simulink model "calculate_thrust"  (R2026a)
settings: Solver=VariableStepAuto
libraries: robotcorelib x1
settings Model: Creator=eqtran103  LastModifiedBy=eqtran103

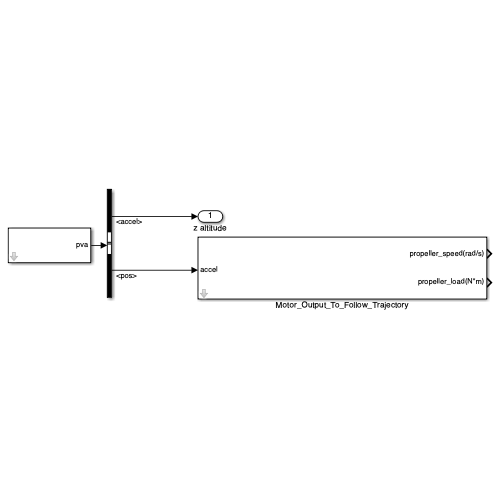
[thumbnail: Simulink's stored preview of the top-level diagram]
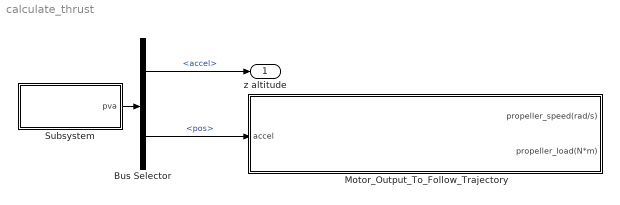
== system calculate_thrust ==
  Bus Selector : BusSelector  OutputSignals=accel,pos
  Motor_Output_To_Follow_Trajectory : Subsystem  mask{Parameter1=0}
  Subsystem : Subsystem  mask{SnapAmplitude=1, JerkCoupleWidth=26.942, TrajectoryTime=100, MaxAccel=1, LaunchTime=10}
  z altitude : Outport
  wires:
  Bus Selector/2 -> Motor_Output_To_Follow_Trajectory/1(accel)  "<pos>"
  Subsystem/1(pva) -> Bus Selector/1
  Bus Selector/1 -> z altitude/1  "<accel>"

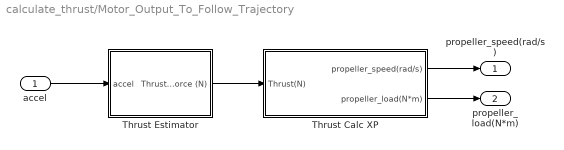
== system calculate_thrust/Motor_Output_To_Follow_Trajectory ==
  accel : Inport
  Thrust Calc XP : Subsystem  mask{L_C=0.02, L_to_D=10}
      mask prompts: L_C "Lift Coefficent (N/(rad/s)^2)"; L_to_D "Lift to Drag (m)"
  Thrust Estimator : Subsystem
  propeller_speed(rad/s) : Outport
  propeller_load(N*m) : Outport  Port=2
  wires:
  Thrust Calc XP/2(propeller_load(N*m)) -> propeller_load(N*m)/1
  accel/1 -> Thrust Estimator/1(accel)
  Thrust Calc XP/1(propeller_speed(rad/s)) -> propeller_speed(rad/s)/1
  Thrust Estimator/1(Thrust_Force (N)) -> Thrust Calc XP/1(Thrust(N))

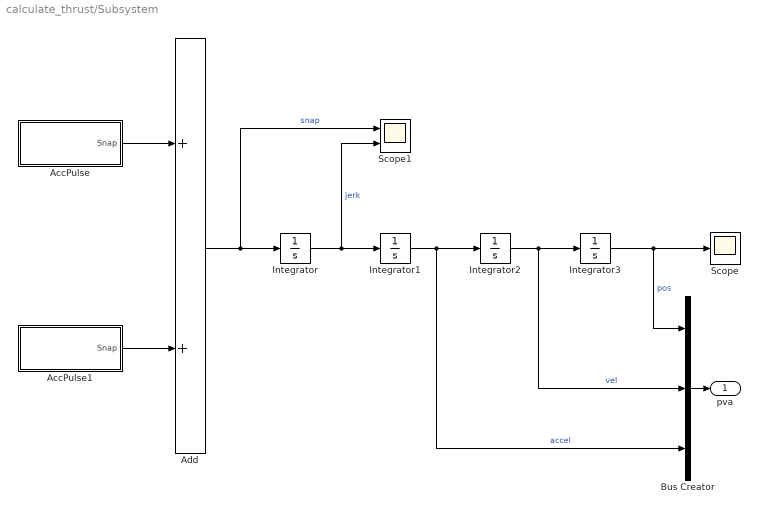
== system calculate_thrust/Subsystem ==
  AccPulse : Subsystem  mask{Amplitude=SnapAmplitude, Width=JerkCoupleWidth, StartTime=LaunchTime}
  AccPulse1 : Subsystem  mask{Amplitude=-SnapAmplitude, Width=JerkCoupleWidth, StartTime=TrajectoryTime - 2*JerkCoupleWidth}
  Add : Sum
  Bus Creator : BusCreator  Inputs=3
  Integrator{,1..3} (4 alike) : Integrator
  Scope : Scope
  Scope1 : Scope  NumInputPorts=2
  pva : Outport
  wires:
  AccPulse/1(Snap) -> Add/1
  AccPulse1/1(Snap) -> Add/2
  Add/1 -> Scope1/1, Integrator/1  "snap"
  Integrator/1 -> Scope1/2, Integrator1/1  "jerk"
  Integrator1/1 -> Bus Creator/3, Integrator2/1  "accel"
  Integrator2/1 -> Bus Creator/2, Integrator3/1  "vel"
  Integrator3/1 -> Bus Creator/1, Scope/1  "pos"
  Bus Creator/1 -> pva/1

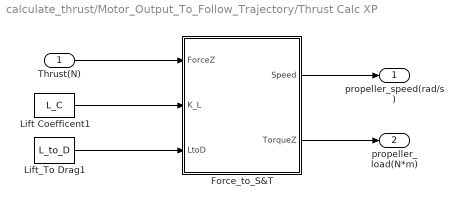
== system calculate_thrust/Motor_Output_To_Follow_Trajectory/Thrust Calc XP ==
  Thrust(N) : Inport
  Force_to_S&T : MATLAB Function  TreatAsAtomicUnit=on
  Lift Coefficent1 : Constant  Value=L_C
  Lift_To Drag1 : Constant  Value=L_to_D
  propeller_speed(rad/s) : Outport
  propeller_load(N*m) : Outport  Port=2
  wires:
  Thrust(N)/1 -> Force_to_S&T/1(ForceZ)
  Lift Coefficent1/1 -> Force_to_S&T/2(K_L)
  Lift_To Drag1/1 -> Force_to_S&T/3(LtoD)
  Force_to_S&T/2(TorqueZ) -> propeller_load(N*m)/1
  Force_to_S&T/1(Speed) -> propeller_speed(rad/s)/1

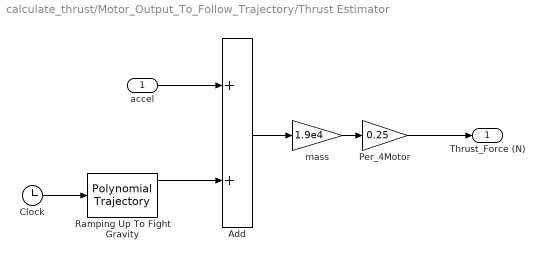
== system calculate_thrust/Motor_Output_To_Follow_Trajectory/Thrust Estimator ==
  accel : Inport
  Add : Sum
  Clock : Clock
  Per_4Motor : Gain  Gain=0.25
  Ramping Up To Fight Gravity : robotcorelib/Polynomial Trajectory  WaypointSource=Internal  Waypoints=[ 0, 9.8]  TimePoints=[ 0, 8]  TimeInterval=[ 1, 4 ]  Method=Cubic Polynomial  ParameterSource=Internal  VelocityBoundaryCondition=zeros( 1, 2 )  AccelerationBoundaryCondition=zeros( 2, 5 )  SimulateUsing=Interpreted execution
  mass : Gain  Gain=1.9e4
  Thrust_Force (N) : Outport
  wires:
  accel/1 -> Add/1
  mass/1 -> Per_4Motor/1
  Add/1 -> mass/1
  Per_4Motor/1 -> Thrust_Force (N)/1
  Clock/1 -> Ramping Up To Fight Gravity/1
  Ramping Up To Fight Gravity/1 -> Add/2

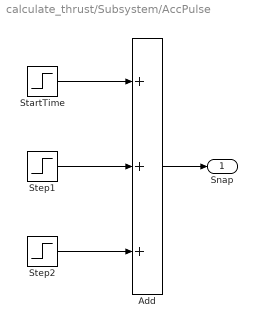
== system calculate_thrust/Subsystem/AccPulse ==
  Add : Sum  Inputs=+++
  StartTime : Step  Time=StartTime  FinalValue=Amplitude  SampleTime=0
  Step1 : Step  Time=StartTime + Width  FinalValue=-2 * Amplitude  SampleTime=0
  Step2 : Step  Time=StartTime + 2*Width  FinalValue=Amplitude  SampleTime=0
  Snap : Outport
  wires:
  Step1/1 -> Add/2
  StartTime/1 -> Add/1
  Step2/1 -> Add/3
  Add/1 -> Snap/1

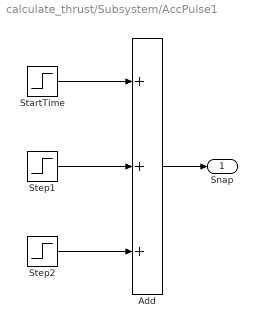
== system calculate_thrust/Subsystem/AccPulse1 ==
  Add : Sum  Inputs=+++
  StartTime : Step  Time=StartTime  FinalValue=Amplitude  SampleTime=0
  Step1 : Step  Time=StartTime + Width  FinalValue=-2 * Amplitude  SampleTime=0
  Step2 : Step  Time=StartTime + 2*Width  FinalValue=Amplitude  SampleTime=0
  Snap : Outport
  wires:
  Step1/1 -> Add/2
  StartTime/1 -> Add/1
  Step2/1 -> Add/3
  Add/1 -> Snap/1

== matlab function calculate_thrust/Motor_Output_To_Follow_Trajectory/Thrust Calc XP/Force_to_S&T ==
  data: Speed output; ForceZ input; TorqueZ output; K_L input; LtoD input
function [Speed, TorqueZ] = fcn(ForceZ, K_L, LtoD)
% ForceZ - desired thrust (from mass*accel + gravity)
% K_L    - lift coefficient gain (speed^2 -> thrust)
% LtoD   - lift-to-drag ratio (thrust -> load torque)
% Speed   - propeller rotational speed required to produce ForceZ
% TorqueZ - resulting load torque on the motor

Speed = sqrt(ForceZ / K_L);
TorqueZ = -ForceZ / LtoD;
end
